simulink model "chatper_8_redo"  (R2024b)
settings: Solver=VariableStepAuto  StartTime=0.0  StopTime=100  RelTol=1e-3
values from neighbouring files (symbols this model uses):
  glide_sys = ss(glide_A,      glide_B,      glide_C,      glide_D, 'StateName',      SS_lo.StateName(glide_states), 'InputName',      SS_lo.InputName(glide_in), 'Name', 'F16 Glide Slope Hold Mode')    [ali_glidslope.m]
  k_q_cas = -0.10753    [ali_glidslope.m]
  theta_gamma = minreal(1 - minreal(delta_e_theta) / minreal(delta_e_alpha))    [ali_glidslope.m]
  trim_state_glide = nan(7,1)    [ali_glidslope.m]
libraries: F16_Actuator_Library x2, slpidlib x2
settings Model: Creator=alial  LastModifiedBy=alial

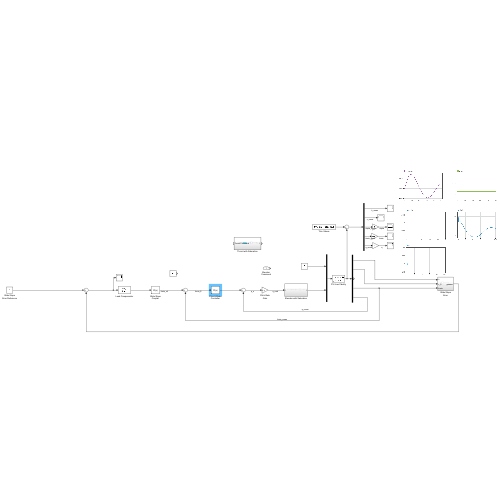
[thumbnail: Simulink's stored preview of the top-level diagram]
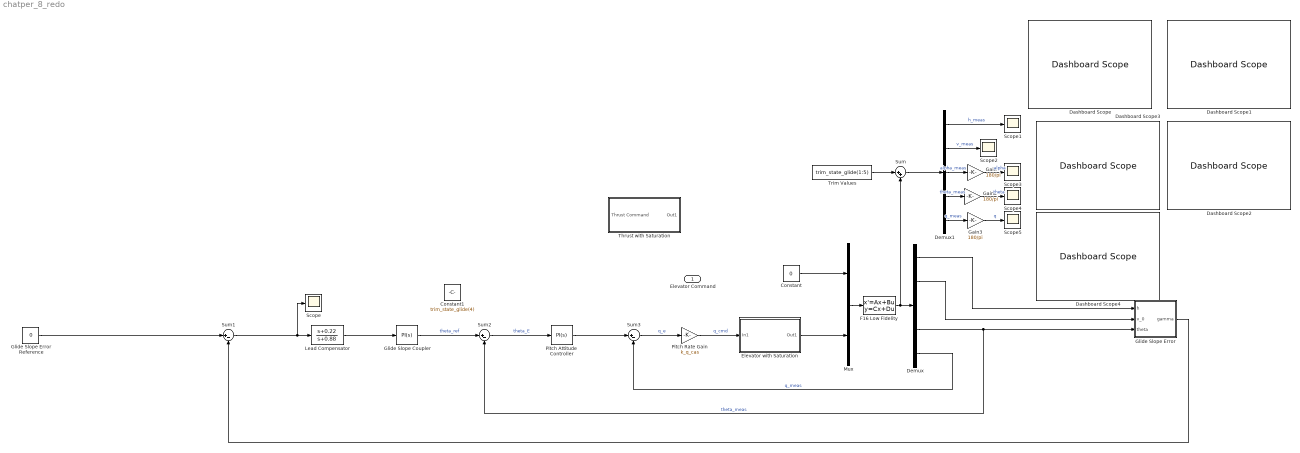
== system chatper_8_redo ==
  Elevator Command : Inport
  Constant : Constant  Value=0
  Constant1 : Constant  Value=trim_state_glide(4)
  Dashboard Scope{,1..4} (5 alike) : DashboardScope
  Demux : Demux  Outputs=[1 1 1 1 1]
  Demux1 : Demux  Outputs=[1 1 1 1 1]
  Elevator with Saturation : Subsystem
  F16 Low Fidelity : StateSpace  A=glide_sys.A  B=glide_sys.B  C=glide_sys.C  D=glide_sys.D  InitialCondition=0  ContinuousStateAttributes=glide_sys.StateName(:)
  Gain : Gain  Gain=180/pi
  Gain2 : Gain  Gain=180/pi
  Gain3 : Gain  Gain=180/pi
  Glide Slope Coupler : slpidlib/PID Controller  Controller=PI  Form=Parallel  TimeDomain=Continuous-time  UseExternalTs=off  SampleTime=-1  IntegratorMethod=Forward Euler  FilterMethod=Forward Euler  ControllerParametersSource=internal  P=-3.99533335724152  I=-0.00653172053613997  UseKiTs=off  D=0  UseExternalDerivativeSource=off  N=100  UseFilter=on  TunerSelectOption=Transfer Function Based (PID Tuner App)  InitialConditionSource=internal  InitialConditionForIntegrator=0  InitialConditionForFilter=0  DifferentiatorICPrevScaledInput=0  ExternalReset=none  TrackingMode=off  Kt=1  LimitOutput=off  SatLimitsSource=internal  UpperSaturationLimit=inf  LowerSaturationLimit=-inf  LinearizeAsGain=on  AntiWindupMode=none  Kb=1  LimitIntegrator=off  UpperIntegratorSaturationLimit=inf  LowerIntegratorSaturationLimit=-inf  POutMin=[]  POutMax=[]  IOutMin=[]  IOutMax=[]  DOutMin=[]  DOutMax=[]  NOutMin=[]  NOutMax=[]  SumOutMin=[]  SumOutMax=[]  SaturationOutMin=[]  SaturationOutMax=[]  PParamMin=[]  PParamMax=[]  IParamMin=[]  IParamMax=[]  DParamMin=[]  DParamMax=[]  NParamMin=[]  NParamMax=[]  KbParamMin=[]  KbParamMax=[]  KtParamMin=[]  KtParamMax=[]  KbOutMin=[]  KbOutMax=[]  KtOutMin=[]  KtOutMax=[]  IntegratorOutMin=[]  IntegratorOutMax=[]  FilterOutMin=[]  FilterOutMax=[]  SumI1OutMin=[]  SumI1OutMax=[]  SumI2OutMin=[]  SumI2OutMax=[]  SumI3OutMin=[]  SumI3OutMax=[]  SumI4OutMin=[]  SumI4OutMax=[]  SumDOutMin=[]  SumDOutMax=[]  DifferentiatorOutMin=[]  DifferentiatorOutMax=[]  FilterDiffOutCoefMin=[]  FilterDiffOutCoefMax=[]  ReciprocalOutMin=[]  ReciprocalOutMax=[]  SumDenOutMin=[]  SumDenOutMax=[]  SumNumOutMin=[]  SumNumOutMax=[]  DivideOutMin=[]  DivideOutMax=[]  UdiffTsProdOutMin=[]  UdiffTsProdOutMax=[]  NTsProdOutMin=[]  NTsProdOutMax=[]  UintegralTsProdOutMin=[]  UintegralTsProdOutMax=[]  UngainTsProdOutMin=[]  UngainTsProdOutMax=[]  ClampingZeroOutDataTypeStr=Inherit: Inherit via back propagation  ClampingZeroOutMin=[]  ClampingZeroOutMax=[]  FilterDenConstantOutDataTypeStr=Inherit: Inherit via back propagation  FilterDenConstantOutMin=[]  FilterDenConstantOutMax=[]  PCopyOutDataTypeStr=Inherit: Inherit via back propagation  PCopyOutMin=[]  PCopyOutMax=[]  NCopyOutDataTypeStr=Inherit: Inherit via back propagation  NCopyOutMin=[]  NCopyOutMax=[]  IntegratorContinuousStateAttributes=''  IntegratorStateMustResolveToSignalObject=off  IntegratorRTWStateStorageClass=Auto  FilterContinuousStateAttributes=''  FilterStateMustResolveToSignalObject=off  FilterRTWStateStorageClass=Auto  ParallelPVariant=InternalParameters  IdealPVariant=Disabled  IVariant=InternalParameters  DVariant=Disabled  IntegratorVariant=Continuous  SatVariant=Disabled  AWVariant=Passthrough  PCopyVariant=Disabled  TRVariant=Disabled  FdbkBlocksVariant=Forward  IdealPFdbkVariant=Disabled  SatFdbkVariant=Disabled  DerivativeFilterVariant=Disabled  NVariant=Disabled  NCopyVariant=Disabled_SignalSpec  FilterICVariant=Disabled  IntegratorICVariant=InternalICs  ExternalResetVariant=Disabled  TRSumVariant=Passthrough  SumFdbkVariant=Disabled  SumVariant=Sum_PI  TsampFilterVariant=InternalTs  TsampNgainVariant=Passthrough  TsampIntegralVariant=Disabled_SignalSpec  ExternalSaturationOutDataTypeStr=Inherit: Same as second input  DerivativeSourceVariant=Disabled  PreIntVariant=InternalPreInt
  Glide Slope Error : Subsystem
  Glide Slope Error Reference : Constant  Value=0
  Lead Compensator : TransferFcn  Numerator=[1 0.22]  Denominator=[1 0.88]
  Mux : Mux  Inputs=2
  Pitch Attitude Controller : slpidlib/PID Controller  Controller=PI  Form=Parallel  TimeDomain=Continuous-time  UseExternalTs=off  SampleTime=-1  IntegratorMethod=Forward Euler  FilterMethod=Forward Euler  ControllerParametersSource=internal  P=0.00698669530728842  I=0.00233198011799084  UseKiTs=off  D=0  UseExternalDerivativeSource=off  N=100  UseFilter=on  TunerSelectOption=Transfer Function Based (PID Tuner App)  InitialConditionSource=internal  InitialConditionForIntegrator=0  InitialConditionForFilter=0  DifferentiatorICPrevScaledInput=0  ExternalReset=none  TrackingMode=off  Kt=1  LimitOutput=off  SatLimitsSource=internal  UpperSaturationLimit=inf  LowerSaturationLimit=-inf  LinearizeAsGain=on  AntiWindupMode=none  Kb=1  LimitIntegrator=off  UpperIntegratorSaturationLimit=inf  LowerIntegratorSaturationLimit=-inf  POutMin=[]  POutMax=[]  IOutMin=[]  IOutMax=[]  DOutMin=[]  DOutMax=[]  NOutMin=[]  NOutMax=[]  SumOutMin=[]  SumOutMax=[]  SaturationOutMin=[]  SaturationOutMax=[]  PParamMin=[]  PParamMax=[]  IParamMin=[]  IParamMax=[]  DParamMin=[]  DParamMax=[]  NParamMin=[]  NParamMax=[]  KbParamMin=[]  KbParamMax=[]  KtParamMin=[]  KtParamMax=[]  KbOutMin=[]  KbOutMax=[]  KtOutMin=[]  KtOutMax=[]  IntegratorOutMin=[]  IntegratorOutMax=[]  FilterOutMin=[]  FilterOutMax=[]  SumI1OutMin=[]  SumI1OutMax=[]  SumI2OutMin=[]  SumI2OutMax=[]  SumI3OutMin=[]  SumI3OutMax=[]  SumI4OutMin=[]  SumI4OutMax=[]  SumDOutMin=[]  SumDOutMax=[]  DifferentiatorOutMin=[]  DifferentiatorOutMax=[]  FilterDiffOutCoefMin=[]  FilterDiffOutCoefMax=[]  ReciprocalOutMin=[]  ReciprocalOutMax=[]  SumDenOutMin=[]  SumDenOutMax=[]  SumNumOutMin=[]  SumNumOutMax=[]  DivideOutMin=[]  DivideOutMax=[]  UdiffTsProdOutMin=[]  UdiffTsProdOutMax=[]  NTsProdOutMin=[]  NTsProdOutMax=[]  UintegralTsProdOutMin=[]  UintegralTsProdOutMax=[]  UngainTsProdOutMin=[]  UngainTsProdOutMax=[]  ClampingZeroOutDataTypeStr=Inherit: Inherit via back propagation  ClampingZeroOutMin=[]  ClampingZeroOutMax=[]  FilterDenConstantOutDataTypeStr=Inherit: Inherit via back propagation  FilterDenConstantOutMin=[]  FilterDenConstantOutMax=[]  PCopyOutDataTypeStr=Inherit: Inherit via back propagation  PCopyOutMin=[]  PCopyOutMax=[]  NCopyOutDataTypeStr=Inherit: Inherit via back propagation  NCopyOutMin=[]  NCopyOutMax=[]  IntegratorContinuousStateAttributes=''  IntegratorStateMustResolveToSignalObject=off  IntegratorRTWStateStorageClass=Auto  FilterContinuousStateAttributes=''  FilterStateMustResolveToSignalObject=off  FilterRTWStateStorageClass=Auto  ParallelPVariant=InternalParameters  IdealPVariant=Disabled  IVariant=InternalParameters  DVariant=Disabled  IntegratorVariant=Continuous  SatVariant=Disabled  AWVariant=Passthrough  PCopyVariant=Disabled  TRVariant=Disabled  FdbkBlocksVariant=Forward  IdealPFdbkVariant=Disabled  SatFdbkVariant=Disabled  DerivativeFilterVariant=Disabled  NVariant=Disabled  NCopyVariant=Disabled_SignalSpec  FilterICVariant=Disabled  IntegratorICVariant=InternalICs  ExternalResetVariant=Disabled  TRSumVariant=Passthrough  SumFdbkVariant=Disabled  SumVariant=Sum_PI  TsampFilterVariant=InternalTs  TsampNgainVariant=Passthrough  TsampIntegralVariant=Disabled_SignalSpec  ExternalSaturationOutDataTypeStr=Inherit: Same as second input  DerivativeSourceVariant=Disabled  PreIntVariant=InternalPreInt
  Pitch Rate Gain : Gain  Gain=k_q_cas
  Scope{,1..5} (6 alike) : Scope
  Sum : Sum  Inputs=|++
  Sum1 : Sum  Inputs=|+-
  Sum2 : Sum  Inputs=|+-
  Sum3 : Sum  Inputs=|+-
  Thrust with Saturation : Subsystem
  Trim Values : Constant  Value=trim_state_glide(1:5)
  wires:
  Glide Slope Error Reference/1 -> Sum1/1
  F16 Low Fidelity/1 -> Demux/1, Sum/2
  Demux/2 -> Glide Slope Error/2(v_0)
  Glide Slope Error/1(gamma) -> Sum1/2
  Mux/1 -> F16 Low Fidelity/1
  Demux/1 -> Glide Slope Error/1(h)
  Pitch Rate Gain/1 -> Elevator with Saturation/1(In1)  "q_cmd"
  Elevator with Saturation/1(Out1) -> Mux/2
  Constant/1 -> Mux/1
  Demux/5 -> Sum3/2  "q_meas"
  Demux/4 -> Sum2/2, Glide Slope Error/3(theta)  "theta_meas"
  Sum3/1 -> Pitch Rate Gain/1  "q_e"
  Trim Values/1 -> Sum/1
  Sum/1 -> Demux1/1
  Sum1/1 -> Scope/1, Lead Compensator/1
  Lead Compensator/1 -> Glide Slope Coupler/1
  Glide Slope Coupler/1 -> Sum2/1  "theta_ref"
  Demux1/1 -> Scope1/1  "h_meas"
  Demux1/2 -> Scope2/1  "v_meas"
  Demux1/5 -> Gain3/1  "q_meas"
  Demux1/4 -> Gain2/1  "theta_meas"
  Demux1/3 -> Gain/1  "alpha_meas"
  Gain/1 -> Scope3/1  "alpha"
  Gain2/1 -> Scope4/1  "theta"
  Gain3/1 -> Scope5/1  "q"
  Pitch Attitude Controller/1 -> Sum3/1
  Sum2/1 -> Pitch Attitude Controller/1  "theta_E"

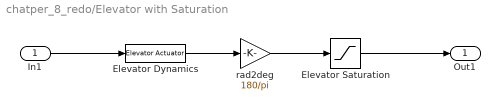
== system chatper_8_redo/Elevator with Saturation ==
  In1 : Inport
  Elevator Dynamics : F16_Actuator_Library/Elevator Actuator  SystemSampleTime=-1  VariantActivationTime=update diagram  AllowFlexibleInterface=on  Latency=0  AutoFrameSizeCalculation=off
  Elevator Saturation : Saturate  UpperLimit=25  LowerLimit=-25
  rad2deg : Gain  Gain=180/pi
  Out1 : Outport
  wires:
  In1/1 -> Elevator Dynamics/1
  Elevator Saturation/1 -> Out1/1
  Elevator Dynamics/1 -> rad2deg/1
  rad2deg/1 -> Elevator Saturation/1

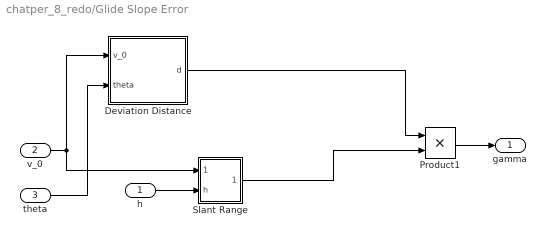
== system chatper_8_redo/Glide Slope Error ==
  h : Inport
  v_0 : Inport  Port=2
  theta : Inport  Port=3
  Deviation Distance : Subsystem
  Product1 : Product
  Slant Range : Subsystem
  gamma : Outport
  wires:
  v_0/1 -> Slant Range/1(v_0), Deviation Distance/1(v_0)
  theta/1 -> Deviation Distance/2(theta)
  Product1/1 -> gamma/1
  Deviation Distance/1(d) -> Product1/1
  h/1 -> Slant Range/2(h)
  Slant Range/1(1/R) -> Product1/2

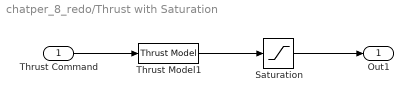
== system chatper_8_redo/Thrust with Saturation ==
  Thrust Command : Inport
  Saturation : Saturate  UpperLimit=19000  LowerLimit=1000
  Thrust Model1 : F16_Actuator_Library/Thrust Model  SystemSampleTime=-1  VariantActivationTime=update diagram  AllowFlexibleInterface=on  Latency=0  AutoFrameSizeCalculation=off
  Out1 : Outport
  wires:
  Thrust Model1/1 -> Saturation/1
  Saturation/1 -> Out1/1
  Thrust Command/1 -> Thrust Model1/1

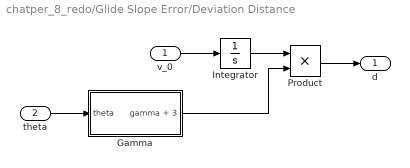
== system chatper_8_redo/Glide Slope Error/Deviation Distance ==
  v_0 : Inport
  theta : Inport  Port=2
  Gamma : Subsystem
  Integrator : Integrator  InitialCondition=trim_state_glide(2)
  Product : Product
  d : Outport
  wires:
  v_0/1 -> Integrator/1
  theta/1 -> Gamma/1(theta)
  Product/1 -> d/1
  Integrator/1 -> Product/1
  Gamma/1(gamma + 3) -> Product/2

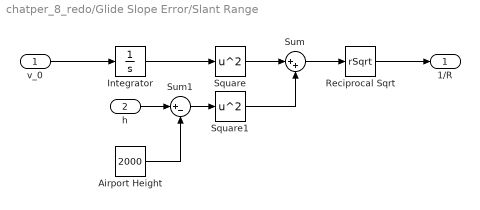
== system chatper_8_redo/Glide Slope Error/Slant Range ==
  v_0 : Inport
  h : Inport  Port=2
  Airport Height : Constant  Value=2000
  Integrator : Integrator
  Reciprocal Sqrt : Sqrt  Operator=rSqrt  IntermediateResultsDataTypeStr=double
  Square : Math  Operator=square
  Square1 : Math  Operator=square
  Sum : Sum  Inputs=|++
  Sum1 : Sum  Inputs=|+-
  1/R : Outport
  wires:
  Square1/1 -> Sum/2
  Integrator/1 -> Square/1
  Airport Height/1 -> Sum1/2
  Sum/1 -> Reciprocal Sqrt/1
  Square/1 -> Sum/1
  Sum1/1 -> Square1/1
  h/1 -> Sum1/1
  v_0/1 -> Integrator/1
  Reciprocal Sqrt/1 -> 1/R/1

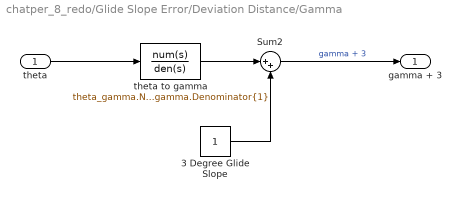
== system chatper_8_redo/Glide Slope Error/Deviation Distance/Gamma ==
  theta : Inport
  3 Degree Glide Slope : Constant
  Sum2 : Sum  Inputs=|++
  theta to gamma : TransferFcn  Numerator=theta_gamma.Numerator{1}  Denominator=theta_gamma.Denominator{1}
  gamma + 3 : Outport
  wires:
  3 Degree Glide Slope/1 -> Sum2/2
  Sum2/1 -> gamma + 3/1  "gamma + 3"
  theta/1 -> theta to gamma/1
  theta to gamma/1 -> Sum2/1
